simulink model "simulink0"  (R2016a)
settings: Solver=ode15s  StartTime=0.0  StopTime=10  RelTol=1e-3
values from neighbouring files (symbols this model uses):
  g = 9.81    [pendulum.m]
  L = 100.0    (= 100)    [pendulum.m]
  theta0 = pi/2    (= 1.57079632679)    [pendulum.m]
  v0 = 0    [pendulum.m]
settings Model: Creator=simone  LastModifiedBy=simone
settings DebuggingCC: AllowedUnitSystems=SI

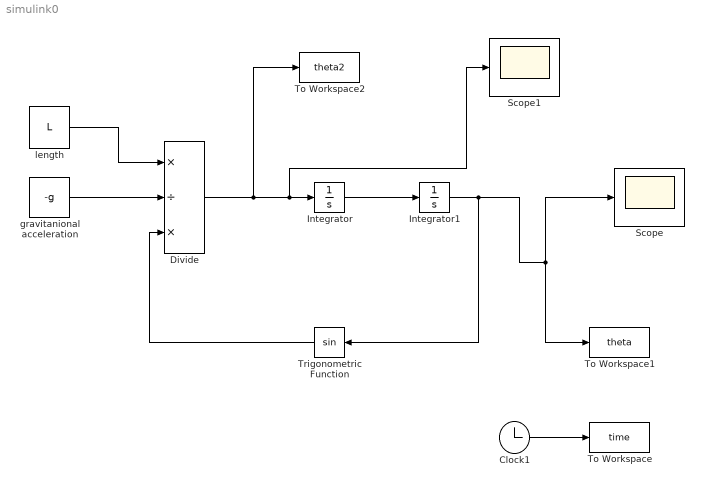
== system simulink0 ==
  Clock1 : Clock
  Divide : Product  Inputs=*/*
  Integrator : Integrator  InitialCondition=v0
  Integrator1 : Integrator  InitialCondition=theta0
  Scope : Scope
  Scope1 : Scope
  To Workspace : ToWorkspace  VariableName=time  SaveFormat=Timeseries  SampleTime=-1
  To Workspace1 : ToWorkspace  VariableName=theta  SaveFormat=Timeseries  SampleTime=-1
  To Workspace2 : ToWorkspace  VariableName=theta2  SaveFormat=Timeseries  SampleTime=-1
  Trigonometric Function : Trigonometry
  gravitanional acceleration : Constant  Value=-g
  length : Constant  Value=L
  wires:
  Integrator/1 -> Integrator1/1
  length/1 -> Divide/1
  gravitanional acceleration/1 -> Divide/2
  Integrator1/1 -> Trigonometric Function/1, To Workspace1/1, Scope/1
  Trigonometric Function/1 -> Divide/3
  Clock1/1 -> To Workspace/1
  Divide/1 -> To Workspace2/1, Scope1/1, Integrator/1
